simulink library "xbsIO"  (Simulink 4.00)
settings Model: Creator=Administrator  LastModifiedBy=haibing

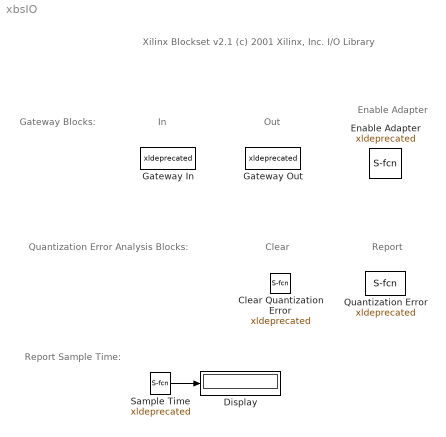
== system xbsIO ==
  note: Xilinx Blockset v2.1
      | (c) 2001 Xilinx, Inc.
      |
      | I/O Library
  note: Quantization Error Analysis Blocks:
  note: Report
  note: Gateway Blocks:
  note: In
  note: Out
  note: Report Sample Time:
  note: Enable Adapter
  note: Clear
  Clear Quantization Error : S-Function  FunctionName=xldeprecated  Parameters=num_inports num_outports  PortCounts=[]  SFunctionModules=''  mask(Xilinx Error Clearing Block){opt_port=off, version=1.1}
      mask prompts: opt_port "Add Optional Clear Port"; version "Version - do not edit"
      mask help: Clear the quantization error tracking mechanism on a trace. Inserting this block will have no effect on the computation outside of error analysis sections. The clear function can also be applied intermittently.
      mask init:
      | num_inports = 1 + opt_port;
      | num_outports = 1;
      | 
      | [bg,fg] = xlcmap('XBlock',1);
      | iPos = get_param(gcb,'Position');
      | iWidth=iPos(3)-iPos(1); iHeight=iPos(4)-iPos(2);
      | iCx=iWidth/2;
      | iCy=iHeight/2;
      | if (opt_port==0)
      |   bg = [1 1 1];
      |   shapeX = iCx* (1 + cos(0:pi/6:2*pi));
      |   shapeY = iCy* (1 + sin(0:pi/6:2*pi));
      |   borderX = [];
      |   borderY = [];
      |   bgX = [];
      |   bgY = [];
      |   pnum=1;
      |   pstr='';
      | else
      |   pnum=2;
      |   pstr='*clrE';
      |   shapeX = .8*iCx* (1.25 + cos(0:pi/6:2*pi));
      |   shapeY = .5*iCy* (2.5 + sin(0:pi/6:2*pi));
      |   borderX = [0 0 iWidth iWidth 0 0 iWidth];
      |   borderY = [0 iHeight iHeight 0 0 0.75*iHeight 0.5*iHeight];
      |   bgX=[0 iWidth iWidth 0];  bgY=[0 0 iHeight iHeight];
      | end
      mask Help: web(xldoclink('Clear Quantization Error'));
      mask Display:
      | patch(bgX,bgY,bg);
      | patch(shapeX,shapeY, [.2 .5 .3]);
      | plot(shapeX,shapeY);
      | plot(borderX, borderY);
      | port_label('input',pnum,pstr);
  Display : Display
      settings: Format=short
      mask Help: web(xldoclink('Display'));
  Enable Adapter : S-Function  Orientation=down  FunctionName=xldeprecated  Parameters=-1 -1  PortCounts=[]  SFunctionModules=''  mask(Xilinx Enable Adapter Block){version=1.1}
      mask prompts: version "Version - do not edit"
      mask help: Adapter block for driving enabled subsystems with the Xilinx fixed point data type.
      mask init:
      | [bg,fg] = xlcmap('IO');
      | iPos = get_param(gcb,'Position');
      | iWidth=iPos(3)-iPos(1); iHeight=iPos(4)-iPos(2);
      | iCx=iWidth/2;
      | iCy=iHeight/2;
      | [logoX, logoY] = xlogo(iPos);
      mask Help: web(xldoclink('Enable Adapter'));
      mask Display:
      | patch([0 iWidth iWidth 0],[0 0 iHeight iHeight] , bg);
      | patch(logoX,logoY , fg);
      | plot([.32*iWidth .42*iWidth .42*iWidth .58*iWidth .58*iWidth .68*iWidth ],[.45*iHeight .45*iHeight .7*iHeight .7*iHeight .45*iHeight .45*iHeight])
      | ;plot([0 0 iWidth iWidth 0], [0 iHeight iHeight 0 0]);
  Gateway In : S-Function  FunctionName=xldeprecated  Parameters=-1 -1  PortCounts=[]  SFunctionModules=''  mask(Xilinx Gateway In Block){arith_type=Signed  (2's comp), n_bits=8, bin_pt=2, quantization=Truncate, overflow=Wrap, period=1, dbl_ovrd=off, timing_constraint=None, locs_specified=off, LOCs={}}
      mask prompts: arith_type "Output Data Type"; n_bits "Number of Bits"; bin_pt "Binary Point"; period "Sample Period"; dbl_ovrd "Override output with double"; timing_constraint "IOB Timing Constraint"; locs_specified "Specify IOB Location Constraints"; LOCs "IOB Pad Locations, e.g.,  {'Valid Bit', 'MSB', ..., 'LSB'}"
      mask help: Gateway in block for the Xilinx Block Set. Converts 'double' type inputs to the Xilinx Fixed point type. In the hardware description, these blocks become top level input ports.
      mask init:
      | dbl_ovrd = xlDblOvrdState(gcb);
      | [bg,fg] = xlcmap('IO',dbl_ovrd);
      | iPos = get_param(gcb,'Position');
      | iWidth=iPos(3)-iPos(1); iHeight=iPos(4)-iPos(2);
      | iCx=iWidth/2;
      | iCy=iHeight/2;
      | [logoX, logoY] = xlogo(iPos);
      mask Help: web(xldoclink('Gateway In'));
      mask StyleString: popup(Unsigned|Signed  (2's comp)),edit,edit,popup(Truncate|Round  (unbiased: +/- Inf)),popup(Wrap|Saturate|Flag as Error),edit,checkbox,popup(None|Data Rate|Data Rate;  Set 'FAST' Attribute),checkbox,edit
      mask Display:
      | patch([0 iWidth iWidth 0],[0 0 iHeight iHeight] , bg);
      | patch(logoX,logoY , fg);
      | port_label('input',1,'dbl');
      | port_label('output',1,'fpt');
      | 
      | ;plot([0 0 iWidth iWidth 0], [0 iHeight iHeight 0 0]);
  Gateway Out : S-Function  FunctionName=xldeprecated  Parameters=-1 -1  PortCounts=[]  SFunctionModules=''  mask(Xilinx Gateway Out Block){hdl_port=on, timing_constraint=None, locs_specified=off, LOCs={}}
      mask prompts: hdl_port "Translate into Output Port"; timing_constraint "IOB Timing Constraint"; locs_specified "Specify IOB Location Constraints"; LOCs "IOB Pad Locations, e.g.,  {'Valid Bit', 'MSB', ..., 'LSB'}"
      mask help: Gateway out block for the Xilinx Block Set. Converts Xilinx Fixed point type inputs into 'double' ouputs. In the hardware description, these blocks can either become top level output ports or be trimmed away, depending on how they are configured.
      mask init:
      | [bg,fg] = xlcmap('IO');
      | if (~hdl_port)
      |   [bg,fg]=xlcmap('XBlock',1);
      | end
      | iPos = get_param(gcb,'Position');
      | iWidth=iPos(3)-iPos(1); iHeight=iPos(4)-iPos(2);
      | iCx=iWidth/2;
      | iCy=iHeight/2;
      | [logoX, logoY] = xlogo(iPos);
      mask Help: web(xldoclink('Gateway Out'));
      mask StyleString: checkbox,popup(None|Data Rate|Data Rate;  Set 'FAST' Attribute),checkbox,edit
      mask Display:
      | patch([0 iWidth iWidth 0],[0 0 iHeight iHeight] , bg);
      | patch(logoX,logoY , fg);
      | port_label('input',1,'fpt');
      | port_label('output',1,'dbl');
      | 
      | ;plot([0 0 iWidth iWidth 0], [0 iHeight iHeight 0 0]);
  Quantization Error : S-Function  FunctionName=xldeprecated  Parameters=-1 -1  PortCounts=[]  SFunctionModules=''  mask(Xilinx Quantization-Error Extractor){version=1.1}
      mask prompts: version "Version - do not edit"
      mask help: Extracts the quantization error from a Xilinx fixed point signal. The quantization error is tracked as the difference between expected value (exact to machine precision) and the actual value represented by the fixed point data.
      mask init:
      | [bg,fg] = xlcmap('IO');
      | iPos = get_param(gcb,'Position');
      | iWidth=iPos(3)-iPos(1); iHeight=iPos(4)-iPos(2);
      | iCx=iWidth/2;
      | iCy=iHeight/2;
      | [logoX, logoY] = xlogo(iPos);
      mask Help: web(xldoclink('Quantization Error'));
      mask Display:
      | patch([0 iWidth iWidth 0],[0 0 iHeight iHeight] , bg);
      | patch(logoX,logoY , fg);
      | port_label('output',1,'err');
      | 
      | ;plot([0 0 iWidth iWidth 0], [0 iHeight iHeight 0 0]);
  Sample Time : S-Function  FunctionName=xldeprecated  Parameters=-1 -1  PortCounts=[]  SFunctionModules=''  mask(Xilinx Sample Time Reporter){version=1.1}
      mask prompts: version "Version - do not edit"
      mask help: Reports the input sample time as a double output.
      mask init:
      | [bg,fg] = xlcmap('IO');
      | iPos = get_param(gcb,'Position');
      | iWidth=iPos(3)-iPos(1); iHeight=iPos(4)-iPos(2);
      | iCx=iWidth/2;
      | iCy=iHeight/2;
      | shapeX = iCx* (1 + cos(0:pi/6:2*pi));
      | shapeY = iCy* (1 + sin(0:pi/6:2*pi));
      mask Help: web(xldoclink('Sample Time'));
      mask Display:
      | patch(shapeX,shapeY, bg);
      | plot(shapeX,shapeY);
      | disp('ST');
  wires:
  Sample Time/1 -> Display/1
